simulink model "gate_V26_2016a"  (R2016a)
settings: Solver=FixedStepDiscrete  StartTime=0.0  StopTime=100  FixedStep=0.001  RelTol=1e-3
undefined symbols (not defined in the file or in its folder): CLOSE_CHAR, CLOSE_SIDE_VALUE, CLOSED, CLOSING, NO_PASS_ASSIG, OPEN, OPEN_CHAR, OPEN_SIDE_VALUE, OPEN_TIMEOUT, OPENING, OPENING_ACTIVE, PASS_ASSIGNED, PASS_INCOMPLETE, PASS_TIMEOUT, PASSWORD_VERIFIED, sigbuilder_block, TIMEOUT, WRONG_PASSWORD
libraries: simulink x9, arduinolib x5
(part 3 of 3)

== stateflow chart gate_V26_2016a/GATE/GATE_B/B_Variant_KP_RF/GateLogicStatemachine ==
  state opening
    entry:
    bulb = true;
    state openLeftSide
      entry:
      leftMotor = OPENING;
      openSideDelay = 0;
      during:
      openSideDelay++;
    state openRightSide
      entry:
      rightMotor = OPENING;
    (default) -> openLeftSide
    openLeftSide -> openRightSide : [openSideDelay == OPEN_SIDE_VALUE]
  state init
    entry:
    passSuccess = NO_PASS_ASSIG;
    gotoReady = false;
    bulb = 0;
    leftMotor = CLOSED;
    rightMotor = CLOSED;
    state AssignPass
      entry:
      counter = 0;
      password[0] = 0;
      password[1] = 0;
      password[2] = 0;
      password[3] = 0;
      password[4] = 0;
      password[5] = 0;
      state addToPass
        entry:
        password[counter] = KpCharPressed;
      state MonitoringNumber
      state PassAssigned
        entry:
        gotoReady = true;
      MonitoringNumber -> (junction 259) [order 1] : [hasChanged(KpCharPressed)]
      (junction 259) -> addToPass : [KpCharPressed != 0]
      (default) -> MonitoringNumber
      addToPass -> MonitoringNumber [order 1] : [counter < 5]/counter++;
      addToPass -> PassAssigned [order 2] : [counter == 5]
          | / passAssigned = true;...
          | passSuccess = PASS_ASSIGNED;
      MonitoringNumber -> PassAssigned [order 2] : [RfOpen == true]
    state idle
      entry:
      passAssigned = false;
    state PassAssignedPreviously
      entry:
      password[0] = passwordIn[0];
      password[1] = passwordIn[1];
      password[2] = passwordIn[2];
      password[3] = passwordIn[3];
      password[4] = passwordIn[4];
      password[5] = passwordIn[5];
      passAssigned = passAssignedIn;
      gotoReady = true;
    (default) -> idle
    idle -> AssignPass [order 1] : [passSwitch==true]
    idle -> PassAssignedPreviously [order 2] : [passAssignedIn]
    AssignPass -> idle : [passSwitch==false]
  state ready
    entry:
    bulb = false;
    leftMotor = CLOSED;
    rightMotor = CLOSED;
    openingActive = 0;
    state openingGate
    state MonitorInput
      entry:
      passTimer = 0;
    state KpPassHandler
      du:
      passTimer++;
      state monitorBtnPressed
      state btnPressed
        entry:
        trialPass[counter] = KpCharPressed;
      state initTrailPass
        entry:
        initCounter = 1;
        state initiatePass
          entry:
          trialPass[initCounter] = 0;
        (junction 269) -> initiatePass
        (default) -> (junction 269)
        initiatePass -> (junction 269) : [initCounter < 5]...
            | /initCounter++;
      state verifyPass
        (default) -> (junction 115)
        (junction 115) -> (junction 116) [order 1] : [trialPass[0] != password[0]]
        (junction 115) -> (junction 119) [order 2]
        (junction 116) -> (junction 118) : {passSuccess = WRONG_PASSWORD;}
        (junction 119) -> (junction 122) [order 1] : [trialPass[1] != password[1]]
        (junction 119) -> (junction 120) [order 2]
        (junction 122) -> (junction 121) : {passSuccess = WRONG_PASSWORD;}
        (junction 120) -> (junction 144) [order 1] : [trialPass[2] != password[2]]
        (junction 120) -> (junction 143) [order 2]
        (junction 144) -> (junction 168) : {passSuccess = WRONG_PASSWORD;}
        (junction 143) -> (junction 149) [order 1] : [trialPass[3] != password[3]]
        (junction 143) -> (junction 153) [order 2]
        (junction 149) -> (junction 169) : {passSuccess = WRONG_PASSWORD;}
        (junction 153) -> (junction 156) [order 1] : [trialPass[4] != password[4]]
        (junction 153) -> (junction 157) [order 2]
        (junction 156) -> (junction 170) : {passSuccess = WRONG_PASSWORD;}
        (junction 157) -> (junction 158) [order 1] : [trialPass[5] != password[5]]
        (junction 157) -> (junction 164) [order 2] : {passSuccess = PASSWORD_VERIFIED;}
        (junction 158) -> (junction 171) : {passSuccess = WRONG_PASSWORD;}
        (junction 171) -> (junction 164)
        (junction 170) -> (junction 171)
        (junction 169) -> (junction 170)
        (junction 168) -> (junction 169)
        (junction 121) -> (junction 168)
        (junction 118) -> (junction 121)
        (junction 164) -> (junction 165)
      (default) -> initTrailPass
      monitorBtnPressed -> (junction 263) : [hasChanged...
          | (KpCharPressed)]
      (junction 263) -> btnPressed : [KpCharPressed != 0]/{counter++;}
      initTrailPass -> monitorBtnPressed : [initCounter == 5]...
          | /{counter = 0;}
      btnPressed -> monitorBtnPressed [order 1] : [counter < 5]
      (junction 262) -> initTrailPass : [(KpCharPressed == OPEN_CHAR)...
          |  && (KpCharPressed != 0)]...
          |  / {openingActive = OPENING_ACTIVE;}
      btnPressed -> verifyPass [order 2] : [counter >= 5]
      verifyPass -> (junction 262) : [hasChanged(KpCharPressed) && (passSuccess == PASSWORD_VERIFIED)]
    (default) -> MonitorInput
    MonitorInput -> openingGate [order 1] : [RfOpen]/{openingActive = OPENING_ACTIVE;}
    KpPassHandler -> MonitorInput [order 3] : [(passTimer == PASS_TIMEOUT)]
        | /passSuccess = TIMEOUT;
    KpPassHandler -> openingGate [order 1] : [openingActive == OPENING_ACTIVE]
    MonitorInput -> (junction 260) [order 2] : [hasChanged...
        | (KpCharPressed)]
    KpPassHandler -> MonitorInput [order 2] : [(passSuccess == WRONG_PASSWORD)]
    (junction 260) -> KpPassHandler : [(KpCharPressed != 0) ...
        | &&(KpCharPressed != OPEN_CHAR)...
        | &&(KpCharPressed != CLOSE_CHAR)...
        | && passAssigned]
        | /passSuccess = PASS_INCOMPLETE;...
        | trialPass[0] = KpCharPressed;
  state closing
    state closingRightSide
      entry:
      rightMotor = CLOSING;
      closeSideDelay = 0;
      during:
      closeSideDelay++;
    state closingLeftSide
      entry:
      leftMotor = CLOSING;
    (default) -> closingRightSide
    closingRightSide -> closingLeftSide : [closeSideDelay == CLOSE_SIDE_VALUE]
  state open
    state gateOpen
      entry:
      closing_active = false;
      leftMotor = OPEN;
      rightMotor = OPEN;
      openTimer = 0;
      du:
      openTimer++;
    state closing
      entry:
      closing_active = true;
    (default) -> gateOpen
    gateOpen -> (junction 264) [order 1] : [hasChanged(KpCharPressed)]
    (junction 264) -> open.closing : [(KpCharPressed == CLOSE_CHAR)]
    gateOpen -> open.closing [order 2] : [RfClose]
    gateOpen -> open.closing [order 3] : [openTimer == OPEN_TIMEOUT]
  ready -> (junction 258) [order 1] : [hasChanged(passSwitch)]
  (junction 258) -> init : [passSwitch]
  (default) -> init
  init -> ready [order 1] : [gotoReady == true]
  ready -> opening [order 2] : [openingActive == OPENING_ACTIVE]
  init -> ready [order 2] : [RfOpen == true]
  closing -> ready : [(current_sensor == 0)...
      | &&(leftMotor == CLOSING)...
      | &&(rightMotor == CLOSING)]
  opening -> open : [(current_sensor == 0)...
      | && (leftMotor == OPENING)...
      | && (rightMotor == OPENING)]
  open -> closing : [closing_active == true]
  data: KpCharPressed input; RfOpen input; openingActive local uint8; passSwitch input; trialPass local uint8 size=6; counter local uint8; closing_active local uint8; current_sensor input; initCounter local uint8; openSideDelay local uint16; leftMotor output uint8 =0; rightMotor output uint8 =0; bulb output boolean; RfClose input; closeSideDelay local uint16; OPENING_ACTIVE input =2; WRONG_PASSWORD input =1; OPEN_SIDE_VALUE input =20; CLOSE_SIDE_VALUE input =20; OPEN_TIMEOUT input =999999; PASSWORD_VERIFIED input =3; CLOSE_CHAR input =12; OPEN_CHAR input; OPENING input =2; CLOSED input =1; CLOSING input =4; OPEN input =3; passAssigned output boolean; gotoReady local boolean; passSuccess output uint8 =0; NO_PASS_ASSIG input; PASS_ASSIGNED input; PASS_INCOMPLETE input; PASS_TIMEOUT input; passTimer local uint16; TIMEOUT input; openTimer local uint16; password output uint8 size=6; passwordIn input size=6; passAssignedIn input

== stateflow chart gate_V26_2016a/GATE/GATE_B/CurrentFilterSubsystem/10msSmapler ==
  (default) -> (junction 2)
  (junction 2) -> (junction 3) : {counter_1ms++;}
  (junction 3) -> (junction 6) : [counter_1ms == 10]
      | {
      | triggerOn;
      | counter_1ms = 0;
      | }
  data: counter_1ms local double
  events: triggerOn output FUNCTION_CALL_EVENT

== stateflow chart gate_V26_2016a/GATE/GATE_B/CurrentFilterSubsystem/Subsystem/SquareWaveDetector ==
  state Running
    entry:
    counterHigh = 0;
    counterLow= 0;
    currentValue = 1;
    state High
      entry:
      counterLow = 0;
    state Low
      entry:
      counterHigh = 0;
    (default) -> High
    High -> High [order 2] : [CurrentAnalogIn > 1000]
        | /counterHigh++;
    High -> Low [order 1] : [CurrentAnalogIn < 1000]
    Low -> High [order 1] : [CurrentAnalogIn > 1000]
    Low -> Low [order 2] : [CurrentAnalogIn < 1000]
        | /counterLow++
  state Stop
    entry:
    currentValue = 0;
    stableCounter = 0;
    state PosEdge
    state NegEdge
    (default) -> PosEdge
    PosEdge -> NegEdge : [(CurrentAnalogInOld > 1000)...
        |  && (CurrentAnalogIn < 1000)]...
        | /stableCounter += 1;
    NegEdge -> PosEdge : [(CurrentAnalogInOld < 1000)...
        |  && (CurrentAnalogIn > 1000)]...
        | /stableCounter += 1;
  (default) -> Stop
  Stop -> Running : [(CurrentAnalogInOld != CurrentAnalogIn) && stableCounter > 2]
  Running -> Stop : [(counterHigh >= 50)...
      |  || (counterLow >= 50)]
  data: CurrentAnalogIn input; currentValue output uint8; counterHigh local uint16; counterLow local uint16; stableCounter local uint8; CurrentAnalogInOld input

== stateflow chart gate_V26_2016a/GATE/GATE_B/EEPROM/EEPROM_Control ==
  state Idle
  state sendData
    entry:
    readReq = true;
  state Read
    entry:
    readReq = false;
  state write
    entry:
    writeReq = true;
  state clear
    entry:
    clearReq = true;
  Read -> sendData
  sendData -> Idle : [readComplete]/readReq = false;
  clear -> Idle [order 2] : [(hasChanged(passSw))...
      |  && (passSw == false)...
      | && (passAssigned == false)]
      | /clearReq = false;
  Idle -> clear : [(hasChanged(passSw))...
      |  && (passSw == true)]
  (default) -> Read
  write -> Read : [writeComplete]/writeReq = false;
  clear -> write [order 1] : [(hasChanged(passSw))...
      |  && (passSw == false)...
      | && (passAssigned == true)]
      | /clearReq = false;
  data: passSw input; passAssigned input; readComplete input; writeComplete input; clearReq output boolean =false; readReq output boolean =false; writeReq output boolean =false

== stateflow chart gate_V26_2016a/GATE/GATE_C/C_Variant_RF/GateLogicStatemachine ==
  state init
    entry:
    gotoReady = false;
    bulb = 0;
    leftMotor = CLOSED;
    rightMotor = CLOSED;
  state opening
    entry:
    bulb = true;
    state openLeftSide
      entry:
      leftMotor = OPENING;
      openSideDelay = 0;
      during:
      openSideDelay++;
    state openRightSide
      entry:
      rightMotor = OPENING;
    (default) -> openLeftSide
    openLeftSide -> openRightSide : [openSideDelay == OPEN_SIDE_VALUE]
  state ready
    entry:
    bulb = false;
    leftMotor = CLOSED;
    rightMotor = CLOSED;
    openingActive = 0;
    state openingGate
      entry:
      openingActive = OPENING_ACTIVE;
    state MonitorInput
    (default) -> MonitorInput
    MonitorInput -> openingGate [order 1] : [RfOpen]
    MonitorInput -> openingGate [order 2] : [passSwitch == true]
  state closing
    state closingRightSide
      entry:
      rightMotor = CLOSING;
      closeSideDelay = 0;
      during:
      closeSideDelay++;
    state closingLeftSide
      entry:
      leftMotor = CLOSING;
    (default) -> closingRightSide
    closingRightSide -> closingLeftSide : [closeSideDelay == CLOSE_SIDE_VALUE]
  state open
    state gateOpen
      entry:
      closing_active = false;
      leftMotor = OPEN;
      rightMotor = OPEN;
      openTimer = 0;
      du:
      openTimer++;
    state closing
      entry:
      closing_active = true;
    (default) -> gateOpen
    gateOpen -> open.closing [order 3] : [passSwitch == true]
    gateOpen -> open.closing [order 1] : [RfClose]
    gateOpen -> open.closing [order 2] : [openTimer == OPEN_TIMEOUT]
  (default) -> init
  ready -> opening : [openingActive == OPENING_ACTIVE]
  init -> ready
  closing -> ready : [(current_sensor == 0)...
      | &&(leftMotor == CLOSING)...
      | &&(rightMotor == CLOSING)]
  opening -> open : [(current_sensor == 0)...
      | && (leftMotor == OPENING)...
      | && (rightMotor == OPENING)]
  open -> closing : [closing_active == true]
  data: RfOpen input; openingActive local uint8; passSwitch input; closing_active local uint8; current_sensor input; openSideDelay local uint16; leftMotor output uint8 =0; rightMotor output uint8 =0; bulb output boolean; RfClose input; closeSideDelay local uint16; OPENING_ACTIVE input =2; OPEN_SIDE_VALUE input =20; CLOSE_SIDE_VALUE input =20; OPEN_TIMEOUT input =999999; OPENING input =2; CLOSED input =1; CLOSING input =4; OPEN input =3; gotoReady local boolean; openTimer local uint16

== stateflow chart gate_V26_2016a/GATE/GATE_C/C_HardwareOutputWrapper_RF/MotorHandler/MotorsHandler ==
  state MonitorChange
  state UpdatePins
    (default) -> (junction 91) : /* updating motor Pins Switch case */
    (junction 91) -> (junction 92) [order 1] : [(leftMotor == OPENING) && ((rightMotor == CLOSED) || (rightMotor == OPEN))]
    (junction 92) -> (junction 100) : {LeftPin = true;...
        | ComPin = true;...
        | RightPin = false;}
    (junction 91) -> (junction 93) [order 2]
    (junction 93) -> (junction 94) [order 1] : [(leftMotor == CLOSING) && ((rightMotor == CLOSED) || (rightMotor == OPEN))]
    (junction 94) -> (junction 99) : {LeftPin = false;...
        | ComPin = false;...
        |  RightPin = true;}
    (junction 93) -> (junction 95) [order 2]
    (junction 95) -> (junction 96) [order 1] : [(rightMotor == CLOSING) && ((leftMotor == CLOSED) || (leftMotor == OPEN))]
    (junction 96) -> (junction 98) : {LeftPin = true;...
        | ComPin = false;...
        | RightPin = false;}
    (junction 95) -> (junction 102) [order 2]
    (junction 102) -> (junction 103) [order 1] : [(rightMotor == OPENING) && ((leftMotor == CLOSED) || (leftMotor == OPEN))]
    (junction 103) -> (junction 110) : {LeftPin = false;...
        | ComPin = true;...
        | RightPin = true;}
    (junction 102) -> (junction 104) [order 2]
    (junction 104) -> (junction 105) [order 1] : [(rightMotor == OPENING) && (leftMotor == OPENING)]
    (junction 105) -> (junction 111) : {LeftPin = true;...
        | ComPin = true;...
        | RightPin = true;}
    (junction 104) -> (junction 106) [order 2]
    (junction 106) -> (junction 107) [order 1] : [(rightMotor == CLOSING) && (leftMotor == CLOSING)]
    (junction 107) -> (junction 112) : {LeftPin = false;...
        | ComPin = false;...
        | RightPin = false;}
    (junction 106) -> (junction 123) [order 2]
    (junction 123) -> (junction 124) [order 1] : [((rightMotor == CLOSED) || (rightMotor == OPEN)) ...
        | && ((leftMotor == CLOSED) || (leftMotor == OPEN))]
    (junction 123) -> (junction 97) [order 2]
    (junction 124) -> (junction 125) : {LeftPin = false;...
        | ComPin = true;...
        | RightPin = false;}
    (junction 100) -> (junction 99)
    (junction 99) -> (junction 98)
    (junction 98) -> (junction 110)
    (junction 125) -> (junction 97)
    (junction 112) -> (junction 125)
    (junction 111) -> (junction 112)
    (junction 110) -> (junction 111)
    (junction 97) -> (junction 101)
  (default) -> MonitorChange
  UpdatePins -> MonitorChange
  MonitorChange -> UpdatePins : [(leftMotor != oldLeft) ...
      | || (rightMotor != oldRight)...
      | || ((rightMotor == CLOSED) && (leftMotor == CLOSED))]
  data: LeftPin output boolean =false; ComPin output boolean =true; RightPin output boolean =false; leftMotor input; oldLeft input; rightMotor input; oldRight input; CLOSED input; CLOSING input; OPEN input; OPENING input

== stateflow chart gate_V26_2016a/GATE/GATE_A/A_HardwareOutputWrapper_BT_KP_RF/BT_TxHandler/BT_TxHandler ==
  state Idle
    entry:
    BT_TxChar = 0;
  state WrongPass
    entry:
    BT_TxChar = 119;
    counter = 0;
    du:
    counter++;
  state BtInput
  state sendClose
    entry:
    BT_TxChar = 99;
  state sendOpen
    entry:
    BT_TxChar = 98;
  state sendOpening
    entry:
    BT_TxChar = 97;
  (default) -> Idle
  Idle -> (junction 8) : [hasChanged(BTCharReceived)]
  (junction 8) -> BtInput : [BTCharReceived != 0]
  sendClose -> Idle : [leftMotor == CLOSED]
  WrongPass -> Idle : [counter >= 10]
  BtInput -> WrongPass [order 2] : [PassSuccess == WRONG_PASSWORD]
  BtInput -> sendOpening [order 1] : [leftMotor == OPENING]
  sendOpen -> sendClose : [rightMotor == CLOSING]
  sendOpening -> sendOpen : [rightMotor == OPEN]
  data: BTCharReceived input; leftMotor input; rightMotor input; BT_TxChar output uint8; PassSuccess input; CLOSED input; CLOSING input; OPEN input; OPENING input; WRONG_PASSWORD input; counter local uint8

== stateflow chart gate_V26_2016a/GATE/GATE_A/A_HardwareOutputWrapper_BT_KP_RF/LedHandler/LedHandler ==
  state AssigningPass
    en:
    counter = 0;
    state Start
      en:
      yellowLedPin = true;
      greenLedPin = false;
      redLedPin = false;
    state correctPassAssigned
      du:
      counter++;
    state incorrectPassAssigned
      du:
      counter++;
    (default) -> AssigningPass.Start
    AssigningPass.Start -> correctPassAssigned [order 1] : [PassAssigned == true]/greenLedPin = true;
    AssigningPass.Start -> incorrectPassAssigned [order 2] : [(PassSw == false) && (PassAssigned == false)]
        | /redLedPin = true;...
        | yellowLedPin = false;
    correctPassAssigned -> correctPassAssigned : [(hasChanged(PassSw)) ...
        | && (PassSw == false)]
        | /yellowLedPin = false;
  state EnteringPass
    en:
    counter = 0;
    state correctPass
      en:
      yellowLedPin = false;
      greenLedPin = true;
      redLedPin = false;
      du:
      counter++;
    state Start
    state IncorrectPass
      en:
      yellowLedPin = false;
      greenLedPin = false;
      redLedPin = true;
      du:
      counter++;
    EnteringPass.Start -> correctPass [order 1] : [PassSuccess == PASSWORD_VERIFIED]
    (default) -> EnteringPass.Start
    EnteringPass.Start -> IncorrectPass [order 2] : [(PassSuccess == TIMEOUT)...
        |  || (PassSuccess == WRONG_PASSWORD)]
  state Idle
    en:
    yellowLedPin = false;
    greenLedPin = false;
    redLedPin = false;
  state GateOn
    en:
    yellowLedPin = false;
    greenLedPin = true;
    redLedPin = false;
  (default) -> Idle
  EnteringPass -> Idle [order 2] : [PassSuccess == NO_PASS_ASSIG]
  Idle -> AssigningPass [order 1] : [PassSw == true]
  correctPass -> Idle : [counter >= 4800]
  AssigningPass -> Idle [order 1] : [(counter >= 4900)]
  Idle -> EnteringPass [order 2] : [(hasChanged(KpCharPressed)) ...
      | && (KpCharPressed != 0)...
      | && (KpCharPressed != OPEN_CHAR)...
      | && (KpCharPressed != CLOSE_CHAR)...
      | && (PassAssigned == true)]
      | /yellowLedPin = true;
  IncorrectPass -> Idle : [counter >= 4800]
  Idle -> GateOn [order 3] : [(leftMotor == OPENING)...
      |  || (leftMotor == OPEN)...
      |  || (leftMotor == CLOSING)]
  GateOn -> Idle : [leftMotor == CLOSED]
  EnteringPass -> GateOn [order 1] : [(leftMotor == OPENING)...
      | || (leftMotor == OPEN)...
      | || (leftMotor == CLOSING)]
  AssigningPass -> GateOn [order 2] : [(leftMotor == OPENING)...
      |  || (leftMotor == OPEN)...
      |  || (leftMotor == CLOSING)]
  data: leftMotor input; greenLedPin output boolean =false; redLedPin output boolean =false; yellowLedPin output boolean =false; PassSw input; counter local uint16; PassAssigned input; PassSuccess input; KpCharPressed input; CLOSED input; CLOSING input; OPEN input; OPENING input; WRONG_PASSWORD input; PASSWORD_VERIFIED input; NO_PASS_ASSIG input; OPEN_CHAR input; CLOSE_CHAR input; TIMEOUT input

== stateflow chart gate_V26_2016a/GATE/GATE_A/A_HardwareOutputWrapper_BT_KP_RF/MotorHandler/MotorsHandler ==
  state MonitorChange
  state UpdatePins
    (default) -> (junction 91) : /* updating motor Pins Switch case */
    (junction 91) -> (junction 92) [order 1] : [(leftMotor == OPENING) && ((rightMotor == CLOSED) || (rightMotor == OPEN))]
    (junction 92) -> (junction 100) : {LeftPin = true;...
        | ComPin = true;...
        | RightPin = false;}
    (junction 91) -> (junction 93) [order 2]
    (junction 93) -> (junction 94) [order 1] : [(leftMotor == CLOSING) && ((rightMotor == CLOSED) || (rightMotor == OPEN))]
    (junction 94) -> (junction 99) : {LeftPin = false;...
        | ComPin = false;...
        |  RightPin = true;}
    (junction 93) -> (junction 95) [order 2]
    (junction 95) -> (junction 96) [order 1] : [(rightMotor == CLOSING) && ((leftMotor == CLOSED) || (leftMotor == OPEN))]
    (junction 96) -> (junction 98) : {LeftPin = true;...
        | ComPin = false;...
        | RightPin = false;}
    (junction 95) -> (junction 102) [order 2]
    (junction 102) -> (junction 103) [order 1] : [(rightMotor == OPENING) && ((leftMotor == CLOSED) || (leftMotor == OPEN))]
    (junction 103) -> (junction 110) : {LeftPin = false;...
        | ComPin = true;...
        | RightPin = true;}
    (junction 102) -> (junction 104) [order 2]
    (junction 104) -> (junction 105) [order 1] : [(rightMotor == OPENING) && (leftMotor == OPENING)]
    (junction 105) -> (junction 111) : {LeftPin = true;...
        | ComPin = true;...
        | RightPin = true;}
    (junction 104) -> (junction 106) [order 2]
    (junction 106) -> (junction 107) [order 1] : [(rightMotor == CLOSING) && (leftMotor == CLOSING)]
    (junction 107) -> (junction 112) : {LeftPin = false;...
        | ComPin = false;...
        | RightPin = false;}
    (junction 106) -> (junction 123) [order 2]
    (junction 123) -> (junction 124) [order 1] : [((rightMotor == CLOSED) || (rightMotor == OPEN)) ...
        | && ((leftMotor == CLOSED) || (leftMotor == OPEN))]
    (junction 123) -> (junction 97) [order 2]
    (junction 124) -> (junction 125) : {LeftPin = false;...
        | ComPin = true;...
        | RightPin = false;}
    (junction 100) -> (junction 99)
    (junction 99) -> (junction 98)
    (junction 98) -> (junction 110)
    (junction 125) -> (junction 97)
    (junction 112) -> (junction 125)
    (junction 111) -> (junction 112)
    (junction 110) -> (junction 111)
    (junction 97) -> (junction 101)
  (default) -> MonitorChange
  UpdatePins -> MonitorChange
  MonitorChange -> UpdatePins : [(leftMotor != oldLeft) ...
      | || (rightMotor != oldRight)...
      | || ((rightMotor == CLOSED) && (leftMotor == CLOSED))]
  data: LeftPin output boolean =false; ComPin output boolean =true; RightPin output boolean =false; leftMotor input; oldLeft input; rightMotor input; oldRight input; CLOSED input; CLOSING input; OPEN input; OPENING input

== stateflow chart gate_V26_2016a/GATE/GATE_B/RFHandler/RFHandlerL ==
  state Close
    entry:
    RFOpen = false;
    RFClose = true;
  state RFOff
    entry:
    RFOpen = false;
    RFClose = false;
  state Open
    entry:
    RFOpen = true;
    RFClose = false;
    counter = 0;
    du:
    counter++;
  Close -> RFOff [order 1] : [rightMotor == CLOSED]
  Close -> (junction 11) [order 2] : [hasChanged(btn)]
  (junction 11) -> Close [order 2] : [(btn == 1) ...
      | && ((leftMotor == OPENING)...
      | || (leftMotor == OPEN))]
  (default) -> RFOff
  RFOff -> (junction 11) : [hasChanged(btn)]
  Open -> (junction 11) [order 2] : [hasChanged(btn)]
  (junction 11) -> Open [order 1] : [(btn == 1) ...
      | && ((leftMotor == CLOSING)...
      | || (leftMotor == CLOSED))]
  Open -> RFOff [order 1] : [(counter == 5) ...
      | && ((leftMotor == CLOSING)...
      | || (leftMotor == CLOSED))]
  data: btn input; RFClose output boolean; RFOpen output boolean; leftMotor input; rightMotor input; CLOSED input; CLOSING input; OPEN input; OPENING input; counter local uint8

== stateflow chart gate_V26_2016a/GATE/GATE_C/CurrentFilterSubsystem/10msSmapler ==
  (default) -> (junction 2)
  (junction 2) -> (junction 3) : {counter_1ms++;}
  (junction 3) -> (junction 6) : [counter_1ms == 10]
      | {
      | triggerOn;
      | counter_1ms = 0;
      | }
  data: counter_1ms local double
  events: triggerOn output FUNCTION_CALL_EVENT

== stateflow chart gate_V26_2016a/GATE/GATE_C/CurrentFilterSubsystem/Subsystem/SquareWaveDetector ==
  state Running
    entry:
    counterHigh = 0;
    counterLow= 0;
    currentValue = 1;
    state High
      entry:
      counterLow = 0;
    state Low
      entry:
      counterHigh = 0;
    (default) -> High
    High -> High [order 2] : [CurrentAnalogIn > 1000]
        | /counterHigh++;
    High -> Low [order 1] : [CurrentAnalogIn < 1000]
    Low -> High [order 1] : [CurrentAnalogIn > 1000]
    Low -> Low [order 2] : [CurrentAnalogIn < 1000]
        | /counterLow++
  state Stop
    entry:
    currentValue = 0;
    stableCounter = 0;
    state PosEdge
    state NegEdge
    (default) -> PosEdge
    PosEdge -> NegEdge : [(CurrentAnalogInOld > 1000)...
        |  && (CurrentAnalogIn < 1000)]...
        | /stableCounter += 1;
    NegEdge -> PosEdge : [(CurrentAnalogInOld < 1000)...
        |  && (CurrentAnalogIn > 1000)]...
        | /stableCounter += 1;
  (default) -> Stop
  Stop -> Running : [(CurrentAnalogInOld != CurrentAnalogIn) && stableCounter > 2]
  Running -> Stop : [(counterHigh >= 50)...
      |  || (counterLow >= 50)]
  data: CurrentAnalogIn input; currentValue output uint8; counterHigh local uint16; counterLow local uint16; stableCounter local uint8; CurrentAnalogInOld input

== stateflow chart gate_V26_2016a/GATE/GATE_C/RFHandler/RFHandlerL ==
  state Close
    entry:
    RFOpen = false;
    RFClose = true;
  state RFOff
    entry:
    RFOpen = false;
    RFClose = false;
  state Open
    entry:
    RFOpen = true;
    RFClose = false;
    counter = 0;
    du:
    counter++;
  Close -> RFOff [order 1] : [rightMotor == CLOSED]
  Close -> (junction 11) [order 2] : [hasChanged(btn)]
  (junction 11) -> Close [order 2] : [(btn == 1) ...
      | && ((leftMotor == OPENING)...
      | || (leftMotor == OPEN))]
  (default) -> RFOff
  RFOff -> (junction 11) : [hasChanged(btn)]
  Open -> (junction 11) [order 2] : [hasChanged(btn)]
  (junction 11) -> Open [order 1] : [(btn == 1) ...
      | && ((leftMotor == CLOSING)...
      | || (leftMotor == CLOSED))]
  Open -> RFOff [order 1] : [(counter == 5) ...
      | && ((leftMotor == CLOSING)...
      | || (leftMotor == CLOSED))]
  data: btn input; RFClose output boolean; RFOpen output boolean; leftMotor input; rightMotor input; CLOSED input; CLOSING input; OPEN input; OPENING input; counter local uint8
